simulink model "dcmotor"  (R2019b)
settings: Solver=VariableStepAuto  StartTime=0.0  StopTime=10.0  RelTol=1e-3
values from neighbouring files (symbols this model uses):
  b = 2.61*10^-4    (= 0.000261)    [params.m]
  J_m = 5.62*10^-5    (= 5.62e-05)    [params.m]
  K_e = 0.068    [params.m]
  K_t = 0.068    [params.m]
  L_a = 3*10^-3    (= 0.003)    [params.m]
  R_a = 1.63    [params.m]
  T_mech = i    [params.m]
  V_a = 14.6    [params.m]
settings Model: Creator=Jasper  LastModifiedBy=Jasper

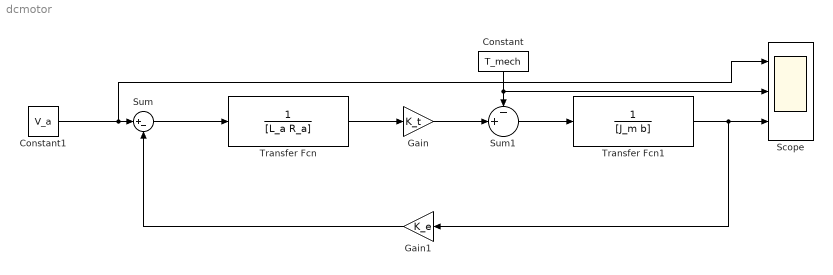
== system dcmotor ==
  Constant : Constant  Value=T_mech
  Constant1 : Constant  Value=V_a
  Gain : Gain  Gain=K_t
  Gain1 : Gain  Gain=K_e
  Scope : Scope  NumInputPorts=3
  Sum : Sum  Inputs=|+-
  Sum1 : Sum  Inputs=-+|
  Transfer Fcn : TransferFcn  Denominator=[L_a R_a]
  Transfer Fcn1 : TransferFcn  Denominator=[J_m b]
  wires:
  Sum/1 -> Transfer Fcn/1
  Transfer Fcn/1 -> Gain/1
  Gain/1 -> Sum1/2
  Constant/1 -> Scope/2, Sum1/1
  Sum1/1 -> Transfer Fcn1/1
  Transfer Fcn1/1 -> Gain1/1, Scope/3
  Constant1/1 -> Scope/1, Sum/1
  Gain1/1 -> Sum/2
